simulink library "GFL_Lib"  (R2020b)
settings: Solver=VariableStepAuto  StartTime=0.0  StopTime=10.0  RelTol=1e-3
values from neighbouring files (symbols this model uses):
  fb = fn    [Init_Base_SM.m]
  Ib2 = Sb / (3*Vb2)    [Init_Base_SM.m]
  Ki_i = Kp_i/Ti_i    [Init_GFL_mod.m]
  Kp_i = 2*zeta_i*wn_i*Lf_pu/wb-Rf_pu    [Init_GFL_mod.m]
  Lb = Zb/wb    [Init_Base_SM.m]
  Lf_pu = Lt_pu    [Init_GFL_mod.m]
  Sb = Pb/cos_phi_n    [Init_Base_SM.m]
  Solver_Time_Step = Time_Step    [Init_LF_L_mod.m]
  Va0 = Vvsc0*sqrt(2)*Vb1*sin(Theta_vsc0*pi/180)    [Init_LF_L_mod.m]
  Vb0 = Vvsc0*sqrt(2)*Vb1*sin(Theta_vsc0*pi/180-2*pi/3)    [Init_LF_L_mod.m]
  Vb1 = Vn1    [Init_Base_SM.m]
  Vb2 = Vn2    [Init_Base_SM.m]
  Vc0 = Vvsc0*sqrt(2)*Vb1*sin(Theta_vsc0*pi/180+2*pi/3)    [Init_LF_L_mod.m]
  Vm0 = abs(V1)    [Init_LF_SM.m]
  Vm0_d = Vvsc0*cos(angle(V1))    [Init_LF_L_mod.m]
  Vm0_q = Vvsc0*sin(angle(V1))    [Init_LF_L_mod.m]
  Vvsc0 = abs(V1)    [Init_LF_L_mod.m]    (also in Init_LF_SM.m = Vm0)
  wb = 2*pi*fb    [Init_Base_SM.m]
  Zb = (3*Vb1^2)/Sb    [Init_Base_SM.m]
undefined symbols (not defined in the file or in its folder): Carm, Diff_CC_ki, Diff_CC_kp, Idcb, Ki_Wdiff_pu, Ki_Wtot_pu, Kp_Rvi_pu, Kp_Wdiff_pu, Kp_Wtot_pu, Lc_eq, Lc_pu, Time_Step, Vdcb, VSC01_id0
libraries: powerlib x90, Control_Lib x57, spsCurrentMeasurementLib x7, spsControlledCurrentSourceLib x6, pid_lib x6, $bdroot x5, Source_Lib x2, eeGeneralControl x2, powerlib_meascontrol x2, simulink x1, GFo_Lib x1
(part 6 of 6)

== system GFL_Lib/Mean Model 2-Level L-filter with DC Link/Control loops/Inner Current Control/Current PI control/PI_fw_init1/Subsystem ==
  e : Inport
  x0 : Inport  Port=2
  Enable : EnablePort
  Integrator : Integrator  InitialConditionSource=external
  y : Outport  VectorParamsAs1DForOutWhenUnconnected=off
  wires:
  x0/1 -> Integrator/2
  Integrator/1 -> y/1
  e/1 -> Integrator/1

== system GFL_Lib/Mean Model 2-Level L-filter_old/Control loops/Inner Current Control/Current PI control/PI_fw_init/Init_condition ==
  y0 : Inport
  comp : Inport  Port=2
  Enable : EnablePort
  Sum : Sum  Inputs=-+
  integ0 : Outport  VectorParamsAs1DForOutWhenUnconnected=off
  wires:
  Sum/1 -> integ0/1
  y0/1 -> Sum/2
  comp/1 -> Sum/1

== system GFL_Lib/Mean Model 2-Level L-filter_old/Control loops/Inner Current Control/Current PI control/PI_fw_init/Subsystem ==
  e : Inport
  x0 : Inport  Port=2
  Enable : EnablePort
  Integrator : Integrator  InitialConditionSource=external
  y : Outport  VectorParamsAs1DForOutWhenUnconnected=off
  wires:
  x0/1 -> Integrator/2
  Integrator/1 -> y/1
  e/1 -> Integrator/1

== system GFL_Lib/Mean Model 2-Level L-filter_old/Control loops/Inner Current Control/Current PI control/PI_fw_init1/Init_condition ==
  y0 : Inport
  comp : Inport  Port=2
  Enable : EnablePort
  Sum : Sum  Inputs=-+
  integ0 : Outport  VectorParamsAs1DForOutWhenUnconnected=off
  wires:
  Sum/1 -> integ0/1
  y0/1 -> Sum/2
  comp/1 -> Sum/1

== system GFL_Lib/Mean Model 2-Level L-filter_old/Control loops/Inner Current Control/Current PI control/PI_fw_init1/Subsystem ==
  e : Inport
  x0 : Inport  Port=2
  Enable : EnablePort
  Integrator : Integrator  InitialConditionSource=external
  y : Outport  VectorParamsAs1DForOutWhenUnconnected=off
  wires:
  x0/1 -> Integrator/2
  Integrator/1 -> y/1
  e/1 -> Integrator/1
